simulink model "adaptive_ModelFollowing"  (R2019b)
settings: Solver=VariableStepAuto  StartTime=0.0  StopTime=60  RelTol=1e-3
values from neighbouring files (symbols this model uses):
  A = [-0.1 2;-2 -0.1]    [EX01a_Linear2D.m]    (also in EX01a_Linear2D_QUANTUM.m = 0*sigma1-2*sigma2+1.5*sigma3-5*sigma4; EX01a_Linear2D_QUANTUM_3.m = A*-j; EX01a_Linear2D_QUANTUM_4.m = A+(basis{i}*rand()); EX01a_Linear2D_QUANTUM_5.m = A+(basis{i}*rand()))
  A_solve = (Xi(1)*sigma1)+(Xi(2)*sigma2)+(Xi(3)*sigma3)+(Xi(4)*sigma4)    [EX01a_Linear2D_QUANTUM.m]    (also in EX01a_Linear2D_QUANTUM_2.m; EX01a_Linear2D_QUANTUM_3.m = A_solve+(Xi(i)*basis{i}*-j); EX01a_Linear2D_QUANTUM_4.m = A_solve+(Xi(i)*basis{i}); EX01a_Linear2D_QUANTUM_5.m = A_solve+(Xi(i)*basis{i}))
settings Model: Creator=tris  LastModifiedBy=tris

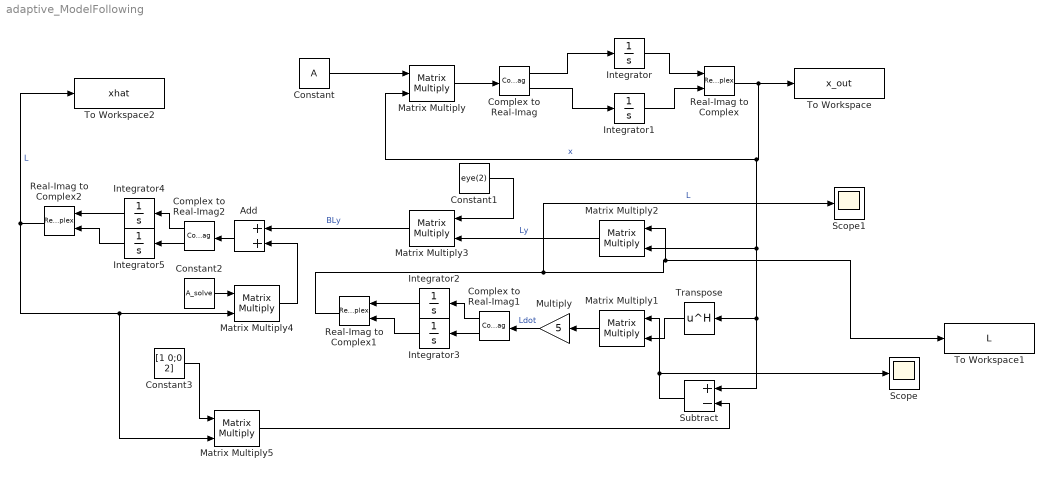
== system adaptive_ModelFollowing ==
  Add : Sum
  Complex to Real-Imag : ComplexToRealImag
  Complex to Real-Imag1 : ComplexToRealImag
  Complex to Real-Imag2 : ComplexToRealImag
  Constant : Constant  Value=A
  Constant1 : Constant  Value=eye(2)
  Constant2 : Constant  Value=A_solve
  Constant3 : Constant  Value=[1 0;0 2]
  Integrator : Integrator  InitialCondition=1
  Integrator{1..5} (5 alike) : Integrator
  Matrix Multiply{,1..5} (6 alike) : Product  Multiplication=Matrix(*)
  Multiply : Gain  Gain=5
  Real-Imag to Complex : RealImagToComplex
  Real-Imag to Complex1 : RealImagToComplex
  Real-Imag to Complex2 : RealImagToComplex
  Scope : Scope
  Scope1 : Scope
  Subtract : Sum  Inputs=+-
  To Workspace : ToWorkspace  VariableName=x_out  SaveFormat=Timeseries  SampleTime=-1
  To Workspace1 : ToWorkspace  VariableName=L  SaveFormat=Timeseries  SampleTime=-1
  To Workspace2 : ToWorkspace  VariableName=xhat  SaveFormat=Timeseries  SampleTime=-1
  Transpose : Math  Operator=hermitian  SignedPower=off  SaturateOnIntegerOverflow=on
  wires:
  Constant/1 -> Matrix Multiply/1
  Matrix Multiply/1 -> Complex to Real-Imag/1
  Complex to Real-Imag/1 -> Integrator/1
  Complex to Real-Imag/2 -> Integrator1/1
  Integrator/1 -> Real-Imag to Complex/1
  Integrator1/1 -> Real-Imag to Complex/2
  Real-Imag to Complex/1 -> To Workspace/1, Matrix Multiply2/2, Subtract/1, Transpose/1, Matrix Multiply/2  "x"
  Matrix Multiply1/1 -> Multiply/1
  Multiply/1 -> Complex to Real-Imag1/1  "Ldot"
  Complex to Real-Imag1/2 -> Integrator3/1
  Complex to Real-Imag1/1 -> Integrator2/1
  Integrator3/1 -> Real-Imag to Complex1/2
  Integrator2/1 -> Real-Imag to Complex1/1
  Real-Imag to Complex1/1 -> Scope1/1, Matrix Multiply2/1, To Workspace1/1  "L"
  Matrix Multiply2/1 -> Matrix Multiply3/2  "Ly"
  Constant1/1 -> Matrix Multiply3/1
  Matrix Multiply3/1 -> Add/1  "BLy"
  Constant2/1 -> Matrix Multiply4/1
  Matrix Multiply4/1 -> Add/2
  Integrator5/1 -> Real-Imag to Complex2/2
  Integrator4/1 -> Real-Imag to Complex2/1
  Complex to Real-Imag2/2 -> Integrator5/1
  Complex to Real-Imag2/1 -> Integrator4/1
  Add/1 -> Complex to Real-Imag2/1
  Real-Imag to Complex2/1 -> Matrix Multiply5/2, Matrix Multiply4/2, To Workspace2/1  "L"
  Transpose/1 -> Matrix Multiply1/2
  Subtract/1 -> Scope/1, Matrix Multiply1/1
  Constant3/1 -> Matrix Multiply5/1
  Matrix Multiply5/1 -> Subtract/2
